simulink model "s_curve"  (R2024b)
settings: Solver=VariableStepAuto  StartTime=0.0  StopTime=10.0  RelTol=1e-3
settings Model: Creator=shohei  LastModifiedBy=shohei

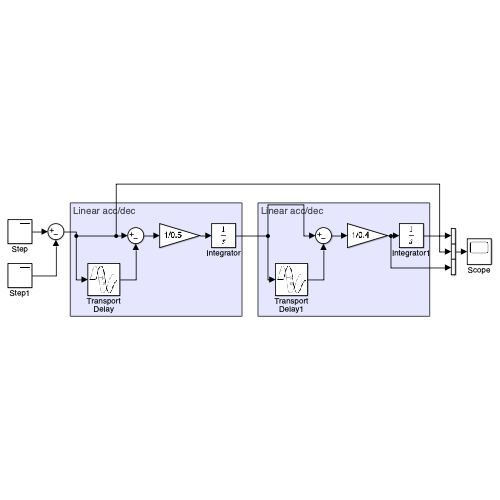
[thumbnail: Simulink's stored preview of the top-level diagram]
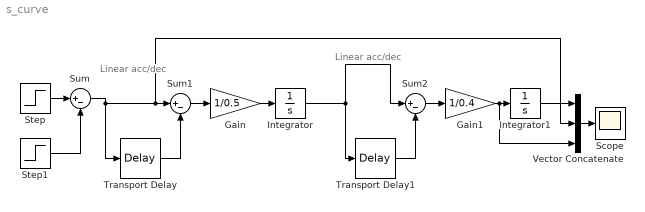
== system s_curve ==
  note: Linear acc/dec
  note: Linear acc/dec
  Gain : Gain  Gain=1/0.5
  Gain1 : Gain  Gain=1/0.4
  Integrator : Integrator
  Integrator1 : Integrator
  Scope : Scope
  Step : Step  SampleTime=0
  Step1 : Step  Time=5  SampleTime=0
  Sum : Sum  Inputs=|+-
  Sum1 : Sum  Inputs=|+-
  Sum2 : Sum  Inputs=|+-
  Transport Delay : TransportDelay  DelayTime=0.5
  Transport Delay1 : TransportDelay  DelayTime=0.4
  Vector Concatenate : Concatenate  NumInputs=3
  wires:
  Transport Delay/1 -> Sum1/2
  Vector Concatenate/1 -> Scope/1
  Sum1/1 -> Gain/1
  Sum/1 -> Vector Concatenate/1, Sum1/1, Transport Delay/1
  Step/1 -> Sum/1
  Step1/1 -> Sum/2
  Gain/1 -> Integrator/1
  Gain1/1 -> Vector Concatenate/3, Integrator1/1
  Transport Delay1/1 -> Sum2/2
  Integrator/1 -> Transport Delay1/1, Sum2/1
  Sum2/1 -> Gain1/1
  Integrator1/1 -> Vector Concatenate/2
